simulink model "HoverAutomate"  (R2020a)
settings: Solver=ode3  StartTime=0.0  StopTime=40  FixedStep=0.001  RelTol=1e-3
model workspace (MAT data in the model file):
  C = 0.0001
  R = 1500
values from neighbouring files (symbols this model uses):
  A = 8.85    [Question3.m]
  T = 2.346    [Question3.m]
settings Model: OrderedModelArguments=off  Creator=shaun  LastModifiedBy=shaun

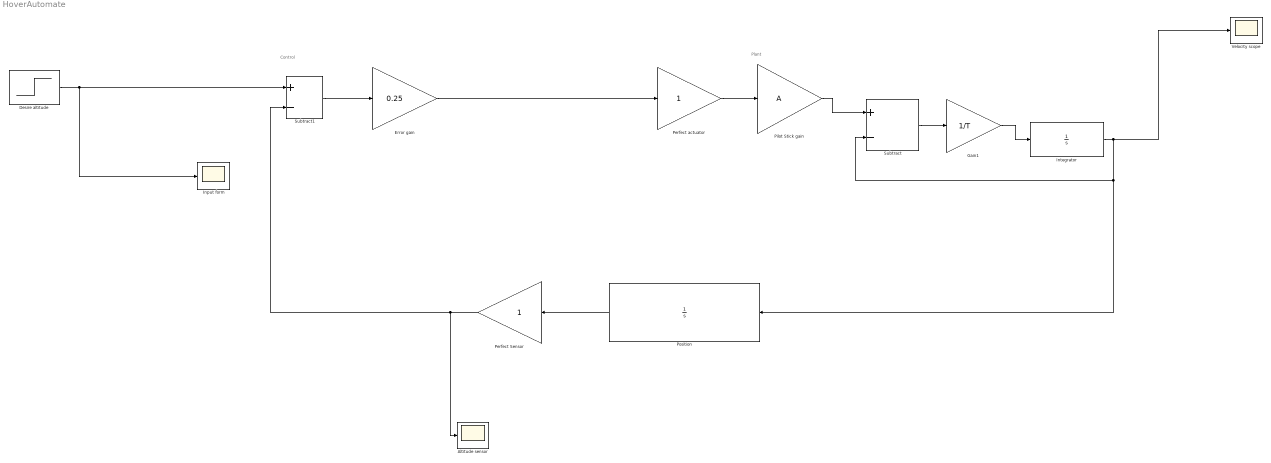
== system HoverAutomate ==
  note: Control
  note: Plant
  " Position" : Integrator
  Altitude sensor : Scope
  Desire altitude : Step  After=13  SampleTime=.05
  Error gain : Gain  Gain=0.25
  Gain1 : Gain  Gain=1/T
  Input form : Scope
  Integrator : Integrator
  Perfect Sensor : Gain
  Perfect actuator : Gain
  Pilot Stick gain : Gain  Gain=A
  Subtract : Sum  Inputs=+-
  Subtract1 : Sum  Inputs=+-
  Velocity scope : Scope
  wires:
  " Position"/1 -> Perfect Sensor/1
  Integrator/1 -> " Position"/1, Subtract/2, Velocity scope/1
  Pilot Stick gain/1 -> Subtract/1
  Gain1/1 -> Integrator/1
  Subtract/1 -> Gain1/1
  Perfect actuator/1 -> Pilot Stick gain/1
  Error gain/1 -> Perfect actuator/1
  Perfect Sensor/1 -> Subtract1/2, Altitude sensor/1
  Desire altitude/1 -> Input form/1, Subtract1/1
  Subtract1/1 -> Error gain/1
